simulink model "odj_sch"  (R2018a)
settings: Solver=VariableStepAuto  StartTime=0.0  StopTime=9000  RelTol=1e-3
values from neighbouring files (symbols this model uses):
  c_p = 1000    [dom_script.m]
  C_vp = c_p*ro_p*V_pp    (= 43200)    [dom_script.m]
  C_vw = c_p*ro_p*V_gp    (= 129600)    [dom_script.m]
  cp = 1000    [odj.m]
  cvp = c_p*ro_p*Vp    [odj.m]
  cvw = c_p*ro_p*Vw    [odj.m]
  d_T = 5    [odj.m]
  d_Tz = -5    [odj.m]
  f_pn = 1    [dom_script.m]
  fp = 1    [odj.m]
  k1 = x(1,1)    [odj.m]
  K_1 = x(1,1)    [dom_script.m]
  K_p = (1/liczba)*K_w    [dom_script.m]
  K_w = x(2,1)    [dom_script.m]
  kp = 0.5*kw    [odj.m]
  kw = x(2,1)    [odj.m]
  ro_p = 1.2    [dom_script.m]
  rop = 1.2    [odj.m]
  steptime = 1    [odj.m]
  T_p_0 = 18    [dom_script.m]
  T_wew_0 = 21    [dom_script.m]
  T_zewn = -1    [dom_script.m]
  T_zn = 24    [dom_script.m]
  Tp0 = Tp    (= 19)    [odj.m]
  Twew = 21    [odj.m]
  Twew0 = Twew    (= 21)    [odj.m]
  Tz = 24    [odj.m]
  Tzew = -4    [odj.m]
settings Model: Creator=jacek  LastModifiedBy=john
settings DataIOCC: ReturnWorkspaceOutputs=on
settings SFSimCC: SimUseLocalCustomCode=on
settings RTWCC: RTWUseLocalCustomCode=on

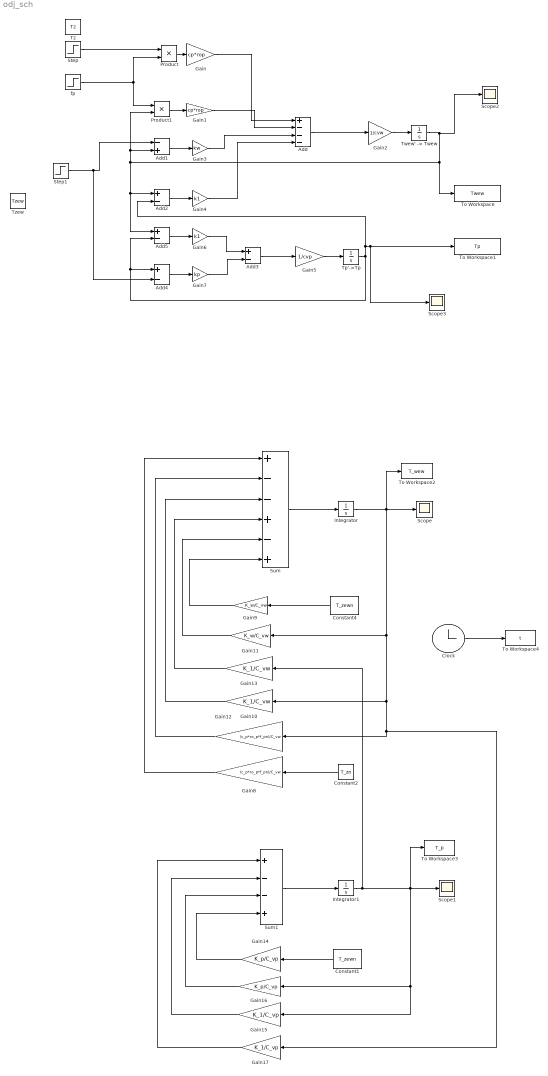
== system odj_sch ==
  Add : Sum  Inputs=+---
  Add1 : Sum  Inputs=-+
  Add{2..5} (4 alike) : Sum  Inputs=+-
  Clock : Clock
  Constant1 : Constant  Value=T_zewn
  Constant2 : Constant  Value=T_zn
  Constant4 : Constant  Value=T_zewn
  Gain : Gain  Gain=cp*rop
  Gain1 : Gain  Gain=cp*rop
  Gain10 : Gain  Gain=K_1/C_vw
  Gain11 : Gain  Gain=K_w/C_vw
  Gain12 : Gain  Gain=(c_p*ro_p*f_pn)/C_vw
  Gain13 : Gain  Gain=K_1/C_vw
  Gain14 : Gain  Gain=K_p/C_vp
  Gain15 : Gain  Gain=K_1/C_vp
  Gain16 : Gain  Gain=K_p/C_vp
  Gain17 : Gain  Gain=K_1/C_vp
  Gain2 : Gain  Gain=1/cvw
  Gain3 : Gain  Gain=kw
  Gain4 : Gain  Gain=k1
  Gain5 : Gain  Gain=1/cvp
  Gain6 : Gain  Gain=k1
  Gain7 : Gain  Gain=kp
  Gain8 : Gain  Gain=(c_p*ro_p*f_pn)/C_vw
  Gain9 : Gain  Gain=K_w/C_vw
  Integrator : Integrator  InitialCondition=T_wew_0
  Integrator1 : Integrator  InitialCondition=T_p_0
  Product : Product
  Product1 : Product
  Scope{,1..3} (4 alike) : Scope
  Step : Step  Time=steptime  Before=Tz  After=Tz+d_Tz  SampleTime=0
  Step1 : Step  Time=steptime  Before=Twew  After=Twew+d_T  SampleTime=0
  Sum : Sum  Inputs=+--+-+
  Sum1 : Sum  Inputs=+--+
  To Workspace : ToWorkspace  VariableName=Twew  SampleTime=-1
  To Workspace1 : ToWorkspace  VariableName=Tp  SampleTime=-1
  To Workspace2 : ToWorkspace  VariableName=T_wew  SaveFormat=Timeseries  SampleTime=-1
  To Workspace3 : ToWorkspace  VariableName=T_p  SaveFormat=Timeseries  SampleTime=-1
  To Workspace4 : ToWorkspace  VariableName=t  SaveFormat=Timeseries  SampleTime=-1
  Tp'->Tp : Integrator  InitialCondition=Tp0
  "Twew' -> Twew" : Integrator  InitialCondition=Twew0
  Tz : Constant  Value=Tz
  Tzew : Constant  Value=Tzew
  fp : Step  Before=fp  After=fp  SampleTime=0
  wires:
  fp/1 -> Product1/1, Product/2
  Product/1 -> Gain/1
  Gain2/1 -> "Twew' -> Twew"/1
  Gain/1 -> Add/1
  Product1/1 -> Gain1/1
  Gain1/1 -> Add/2
  Add1/1 -> Gain3/1
  Gain3/1 -> Add/3
  Add2/1 -> Gain4/1
  Gain4/1 -> Add/4
  Add/1 -> Gain2/1
  "Twew' -> Twew"/1 -> Scope2/1, To Workspace/1, Product1/2, Add1/2, Add5/1, Add2/1
  Gain5/1 -> Tp'->Tp/1
  Add3/1 -> Gain5/1
  Gain6/1 -> Add3/1
  Gain7/1 -> Add3/2
  Add5/1 -> Gain6/1
  Add4/1 -> Gain7/1
  Tp'->Tp/1 -> Scope3/1, To Workspace1/1, Add2/2, Add4/1, Add5/2
  Sum1/1 -> Integrator1/1
  Gain10/1 -> Sum/3
  Constant4/1 -> Gain9/1
  Gain9/1 -> Sum/6
  Gain11/1 -> Sum/5
  Gain8/1 -> Sum/1
  Constant2/1 -> Gain8/1
  Sum/1 -> Integrator/1
  Gain14/1 -> Sum1/4
  Gain16/1 -> Sum1/3
  Gain15/1 -> Sum1/2
  Integrator/1 -> To Workspace2/1, Gain11/1, Gain10/1, Gain17/1, Gain12/1, Scope/1
  Gain17/1 -> Sum1/1
  Gain13/1 -> Sum/4
  Constant1/1 -> Gain14/1
  Integrator1/1 -> To Workspace3/1, Gain15/1, Gain16/1, Scope1/1, Gain13/1
  Clock/1 -> To Workspace4/1
  Gain12/1 -> Sum/2
  Step/1 -> Product/1
  Step1/1 -> Add4/2, Add1/1
